simulink model "modelisland"  (Simulink 9.2)
settings: Solver=ode3  StartTime=0.0  StopTime=2  RelTol=1e-3  EnableMultiTasking=on
libraries: powerlib x11, powerlib_extras x1
settings Model: Creator=pc  LastModifiedBy=HP
settings SolverCC: ZeroCrossAlgorithm=Adaptive
settings OptimizationCC: ExpressionDepthLimit=2147483647
settings DebuggingCC: MaskedZcDiagnostic=none  IgnoredZcDiagnostic=none  SolverPrmCheckMsg=warning

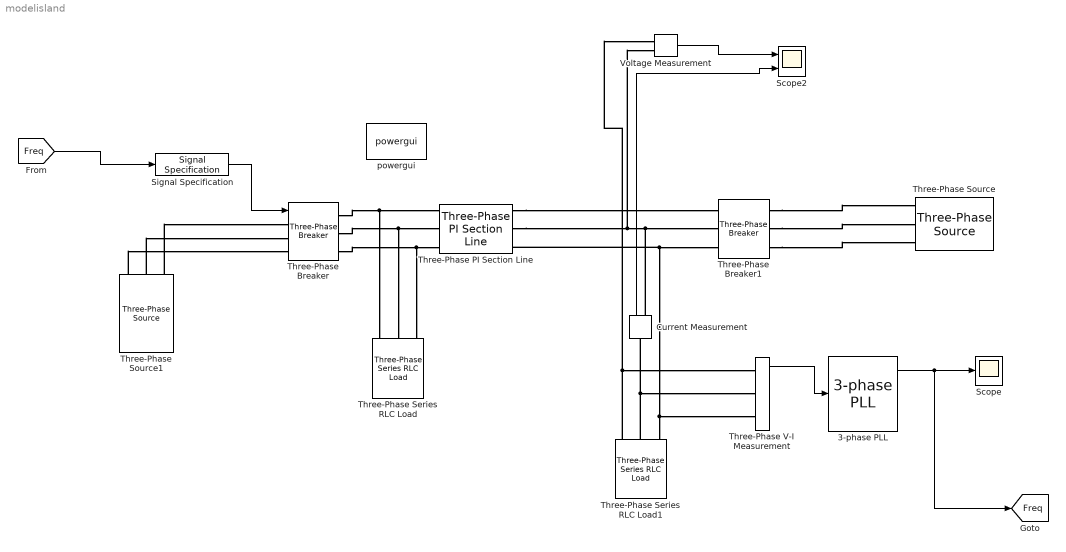
== system modelisland ==
  3-phase PLL : powerlib_extras/Control  Blocks/3-phase PLL  Par_Init=[0 60]  ParK=[ 180 3200 1 ]  AGC=off
  Current Measurement : powerlib/Measurements/Current Measurement  PhasorSimulation=off  OutputType=Complex  PSBequivalent=0
  Scope : Scope
  Scope2 : Scope  NumInputPorts=2
  Signal Specification : SignalSpecification
  Three-Phase PI Section Line : powerlib/Elements/Three-Phase PI Section Line  LConnTagsString=a|b|c  RConnTagsString=A|B|C  Frequency=60  Resistances=[ 0.01273 0.3864]  Inductances="[ 0.9337e-3  4.1264e-3]"  Capacitances=[12.74e-9 7.751e-9]  Length=500
      settings: SourceProductName=Simscape Power Systems
  Three-Phase Series RLC Load : powerlib/Elements/Three-Phase Series RLC Load  LConnTagsString=A|B|C  Configuration=Y (grounded)  NominalVoltage=1000  Vabc=[1e3 1e3 1e3]  Vabcp=[1e3 1e3 1e3]  NominalFrequency=60  UnbalancedPower=off  ActivePower=10e3  InductivePower=100  CapacitivePower=100  Pabc=[10e3 9e3 11e3]  QLabc=[100 90 110]  QCabc=[100 90 110]  Pabcp=[10e3 9e3 11e3]  QLabcp=[100 90 110]  QCabcp=[100 90 110]  Measurements=None  LoadType=constant Z
  Three-Phase Series RLC Load1 : powerlib/Elements/Three-Phase Series RLC Load  LConnTagsString=A|B|C  Configuration=Y (grounded)  NominalVoltage=1000  Vabc=[1e3 1e3 1e3]  Vabcp=[1e3 1e3 1e3]  NominalFrequency=60  UnbalancedPower=off  ActivePower=10e3  InductivePower=100  CapacitivePower=100  Pabc=[10e3 9e3 11e3]  QLabc=[100 90 110]  QCabc=[100 90 110]  Pabcp=[10e3 9e3 11e3]  QLabcp=[100 90 110]  QCabcp=[100 90 110]  Measurements=None  LoadType=constant Z
  Three-Phase V-I Measurement : powerlib/Measurements/Three-Phase V-I Measurement  VoltageMeasurement=phase-to-ground  SetLabelV=off  LabelV=Vabc  Vpu=off  VpuLL=off  CurrentMeasurement=no  SetLabelI=off  LabelI=Iabc  Ipu=off  Pbase=100e6  Vbase=500e3  OutputType=Complex  PhasorSimulation=off  PSBequivalent=0
  Three-Phase Breaker : powerlib/Elements/Three-Phase Breaker  InitialState=closed  SwitchA=on  SwitchB=on  SwitchC=on  SwitchTimes="[4/60  10/60]"  External=on  BreakerResistance=0.001  SnubberResistance=1e6  SnubberCapacitance=inf  Measurements=None
  Three-Phase Breaker1 : powerlib/Elements/Three-Phase Breaker  InitialState=open  SwitchA=on  SwitchB=on  SwitchC=on  SwitchTimes="[4/60  10/60]"  External=off  BreakerResistance=0.001  SnubberResistance=1e6  SnubberCapacitance=inf  Measurements=None
  Three-Phase Source : powerlib/Electrical Sources/Three-Phase Source  InternalConnection=Yg  VoltagePhases=off  Voltage=25e3  PhaseAngle=0  Voltage_phases=[25e3 25e3 25e3]/sqrt(3)  PhaseAngles_phases=[0 -120 +120]  Frequency=60  NonIdealSource=on  SpecifyImpedance=on  Resistance=0.8929  Inductance=16.58e-3  ShortCircuitLevel=100e6  BaseVoltage=25e3  XRratio=7  BusType=swing  Pref=10e3  Qref=0  Prefabc=[10e3, 10e3, 10e3]  Qrefabc=[0, 0, 0]  Qmin=-inf  Qmax=inf
  Three-Phase Source1 : powerlib/Electrical Sources/Three-Phase Source  InternalConnection=Yg  VoltagePhases=off  Voltage=25e3  PhaseAngle=0  Voltage_phases=[25e3 25e3 25e3]/sqrt(3)  PhaseAngles_phases=[0 -120 +120]  Frequency=60  NonIdealSource=on  SpecifyImpedance=on  Resistance=0.8929  Inductance=16.58e-3  ShortCircuitLevel=100e6  BaseVoltage=25e3  XRratio=7  BusType=swing  Pref=10e3  Qref=0  Prefabc=[10e3, 10e3, 10e3]  Qrefabc=[0, 0, 0]  Qmin=-inf  Qmax=inf
  Voltage Measurement : powerlib/Measurements/Voltage Measurement  PhasorSimulation=off  OutputType=Complex  PSBequivalent=0
  powergui : powerlib/powergui  Priority=1  SimulationMode=Discrete  SampleTime=50e-6  frequency=60  Iterations=50  frequencyindice=60  Pbase=100e6  ErrMax=1e-4  UnitsV=kV  UnitsW=MW  buscounter=0  FunctionMessages=off  echomessages=off  EnableUseOfTLC=off  CurrentSourceSwitches=off  DisableSnubberDevices=off  DisableRonSwitches=off  DisableVfSwitches=off  DisplayEquations=off  SolverType=Tustin/Backward Euler (TBE)  Interpol=off  ExternalGateDelay=off  methode=off  Ts=100  x0status=blocks  SPID=off  SwTol=0  HookPort=off  RestoreLinks=warning  ResistiveCurrentMeasurement=off  Frange=[0:2:500]  Ylog=off  Xlog=on  ShowGrid=off  save=off  variable=ZData  structure=0  ZoomFFT=off  StartTime=0.0  cycles=1  DisplayStyle=1  fundamental=60  FreqAxis=off  MaxFrequency=1000  frequencyindicesteady=1  RmsSteady=1  display=off
  tag scope: Freq=global
  wires:
  Current Measurement/1 -> Scope2/2
  Voltage Measurement/1 -> Scope2/1
  Three-Phase V-I Measurement/1 -> 3-phase PLL/1
  Signal Specification/1 -> Three-Phase Breaker/1
  [Freq] -> Signal Specification/1
  3-phase PLL/1 -> Scope/1, [Freq]
  connections:
  Three-Phase Breaker/RConn1 -- Three-Phase PI Section Line/LConn1 -- Three-Phase Series RLC Load/LConn1
  Three-Phase Breaker/RConn2 -- Three-Phase PI Section Line/LConn2 -- Three-Phase Series RLC Load/LConn2
  Three-Phase Breaker/RConn3 -- Three-Phase PI Section Line/LConn3 -- Three-Phase Series RLC Load/LConn3
  Three-Phase PI Section Line/RConn1 -- Three-Phase Breaker1/LConn1
  Three-Phase PI Section Line/RConn2 -- Voltage Measurement/LConn2 -- Three-Phase Breaker1/LConn2 -- Current Measurement/RConn1
  Three-Phase Breaker1/LConn3 -- Three-Phase PI Section Line/RConn3 -- Three-Phase Series RLC Load1/LConn3 -- Three-Phase V-I Measurement/LConn3
  Three-Phase Breaker1/RConn1 -- Three-Phase Source/RConn1
  Three-Phase Breaker1/RConn2 -- Three-Phase Source/RConn2
  Three-Phase Breaker1/RConn3 -- Three-Phase Source/RConn3
  Three-Phase Series RLC Load1/LConn2 -- Current Measurement/LConn1 -- Three-Phase V-I Measurement/LConn2
  Three-Phase Series RLC Load1/LConn1 -- Voltage Measurement/LConn1 -- Three-Phase V-I Measurement/LConn1
  Three-Phase Source1/RConn1 -- Three-Phase Breaker/LConn1
  Three-Phase Source1/RConn2 -- Three-Phase Breaker/LConn2
  Three-Phase Source1/RConn3 -- Three-Phase Breaker/LConn3
